simulink model "case4"  (R2024b)
settings: Solver=FixedStepAuto  StartTime=0  StopTime=1  FixedStep=1e-7  RelTol=1e-3
values from neighbouring files (symbols this model uses):
  SG_D_1_D = 0.01056    [IEEE9_case_parameters.m]    (also in case1_parameters.m; case2_parameters.m; case3_parameters.m; case4_parameters.m)
  SG_D_1_EnableSaturation = 0    [IEEE9_case_parameters.m]    (also in case1_parameters.m; case2_parameters.m; case3_parameters.m; case4_parameters.m)
  SG_D_1_f0 = 60    [IEEE9_case_parameters.m]    (also in case1_parameters.m; case2_parameters.m; case3_parameters.m; case4_parameters.m)
  SG_D_1_H = 7.5    [IEEE9_case_parameters.m]    (also in case1_parameters.m; case2_parameters.m; case3_parameters.m; case4_parameters.m)
  SG_D_1_K_A = 20    [IEEE9_case_parameters.m]    (also in case1_parameters.m; case2_parameters.m; case3_parameters.m; case4_parameters.m)
  SG_D_1_K_E = 1.000000e+1    (= 10)    [IEEE9_case_parameters.m]    (also in case1_parameters.m; case2_parameters.m; case3_parameters.m; case4_parameters.m)
  SG_D_1_K_F = 2.363    [IEEE9_case_parameters.m]    (also in case1_parameters.m; case2_parameters.m; case3_parameters.m; case4_parameters.m)
  SG_D_1_K_s = 0.5    [IEEE9_case_parameters.m]    (also in case1_parameters.m = 5; case2_parameters.m = 5; case3_parameters.m = 5; case4_parameters.m = 5)
  SG_D_1_R_a = 0.001088    [IEEE9_case_parameters.m]    (also in case1_parameters.m; case2_parameters.m; case3_parameters.m; case4_parameters.m)
  SG_D_1_S_A = 1    [IEEE9_case_parameters.m]    (also in case1_parameters.m; case2_parameters.m; case3_parameters.m; case4_parameters.m)
  SG_D_1_S_B = 0.103    [IEEE9_case_parameters.m]    (also in case1_parameters.m; case2_parameters.m; case3_parameters.m; case4_parameters.m)
  SG_D_1_S_N = 10.659857    [IEEE9_case_parameters.m]    (also in case1_parameters.m; case2_parameters.m; case3_parameters.m; case4_parameters.m)
  SG_D_1_SpeedPara = 200    [IEEE9_case_parameters.m]    (also in case1_parameters.m; case2_parameters.m; case3_parameters.m; case4_parameters.m)
  SG_D_1_T_0 = 0.720173    [IEEE9_case_parameters.m]    (also in case1_parameters.m = 0.755522; case2_parameters.m = 0.808931; case3_parameters.m = 0.869402; case4_parameters.m = 0.729316)
  SG_D_1_T_1 = 0.3    [IEEE9_case_parameters.m]    (also in case1_parameters.m; case2_parameters.m; case3_parameters.m; case4_parameters.m)
  SG_D_1_T_2 = 0.05    [IEEE9_case_parameters.m]    (also in case1_parameters.m; case2_parameters.m; case3_parameters.m; case4_parameters.m)
  SG_D_1_T_3 = 0.02    [IEEE9_case_parameters.m]    (also in case1_parameters.m; case2_parameters.m; case3_parameters.m; case4_parameters.m)
  SG_D_1_T_4 = 0.005    [IEEE9_case_parameters.m]    (also in case1_parameters.m; case2_parameters.m; case3_parameters.m; case4_parameters.m)
  SG_D_1_T_A = 0.02    [IEEE9_case_parameters.m]    (also in case1_parameters.m; case2_parameters.m; case3_parameters.m; case4_parameters.m)
  SG_D_1_T_dd = 8.000000e+0    (= 8)    [IEEE9_case_parameters.m]    (also in case1_parameters.m; case2_parameters.m; case3_parameters.m; case4_parameters.m)
  SG_D_1_T_ddd = 0.04    [IEEE9_case_parameters.m]    (also in case1_parameters.m; case2_parameters.m; case3_parameters.m; case4_parameters.m)
  SG_D_1_T_E = 0.314    [IEEE9_case_parameters.m]    (also in case1_parameters.m; case2_parameters.m; case3_parameters.m; case4_parameters.m)
  SG_D_1_T_F = 0.35    [IEEE9_case_parameters.m]    (also in case1_parameters.m; case2_parameters.m; case3_parameters.m; case4_parameters.m)
  SG_D_1_T_qd = 0.8    [IEEE9_case_parameters.m]    (also in case1_parameters.m; case2_parameters.m; case3_parameters.m; case4_parameters.m)
  SG_D_1_T_qdd = 0.02    [IEEE9_case_parameters.m]    (also in case1_parameters.m; case2_parameters.m; case3_parameters.m; case4_parameters.m)
  SG_D_1_T_speed = 0.1    [IEEE9_case_parameters.m]    (also in case1_parameters.m = 200; case2_parameters.m = 200; case3_parameters.m = 200; case4_parameters.m = 200)
  SG_D_1_T_w = 0.5    [IEEE9_case_parameters.m]    (also in case1_parameters.m; case2_parameters.m; case3_parameters.m; case4_parameters.m)
  SG_D_1_V_ref = 1.990276    [IEEE9_case_parameters.m]    (also in case1_parameters.m = 2.042296; case2_parameters.m = 2.051388; case3_parameters.m = 2.089584; case4_parameters.m = 2.01845)
  SG_D_1_w_ref = 376.991118    [IEEE9_case_parameters.m]    (also in case1_parameters.m; case2_parameters.m; case3_parameters.m; case4_parameters.m)
  SG_D_1_wb = 6.000000e+1    (= 60)    [IEEE9_case_parameters.m]    (also in case1_parameters.m; case2_parameters.m; case3_parameters.m; case4_parameters.m)
  SG_D_1_x_d = 1.9    [IEEE9_case_parameters.m]    (also in case1_parameters.m; case2_parameters.m; case3_parameters.m; case4_parameters.m)
  SG_D_1_x_dd = 0.302    [IEEE9_case_parameters.m]    (also in case1_parameters.m; case2_parameters.m; case3_parameters.m; case4_parameters.m)
  SG_D_1_x_ddd = 0.204    [IEEE9_case_parameters.m]    (also in case1_parameters.m; case2_parameters.m; case3_parameters.m; case4_parameters.m)
  SG_D_1_x_l = 0.05    [IEEE9_case_parameters.m]    (also in case1_parameters.m; case2_parameters.m; case3_parameters.m; case4_parameters.m)
  SG_D_1_x_q = 1.3    [IEEE9_case_parameters.m]    (also in case1_parameters.m; case2_parameters.m; case3_parameters.m; case4_parameters.m)
  SG_D_1_x_qd = 0.5    [IEEE9_case_parameters.m]    (also in case1_parameters.m; case2_parameters.m; case3_parameters.m; case4_parameters.m)
  SG_D_1_x_qdd = 0.3    [IEEE9_case_parameters.m]    (also in case1_parameters.m; case2_parameters.m; case3_parameters.m; case4_parameters.m)
  SG_D_2_D = 0.02    [IEEE9_case_parameters.m]    (also in case1_parameters.m; case2_parameters.m; case3_parameters.m; case4_parameters.m)
  SG_D_2_EnableSaturation = 0    [IEEE9_case_parameters.m]    (also in case1_parameters.m; case2_parameters.m; case3_parameters.m; case4_parameters.m)
  SG_D_2_f0 = 60    [IEEE9_case_parameters.m]    (also in case1_parameters.m; case2_parameters.m; case3_parameters.m; case4_parameters.m)
  SG_D_2_H = 8.000000e+0    (= 8)    [IEEE9_case_parameters.m]    (also in case1_parameters.m; case2_parameters.m; case3_parameters.m; case4_parameters.m)
  SG_D_2_K_A = 20    [IEEE9_case_parameters.m]    (also in case1_parameters.m; case2_parameters.m; case3_parameters.m; case4_parameters.m)
  SG_D_2_K_E = 1.000000e+1    (= 10)    [IEEE9_case_parameters.m]    (also in case1_parameters.m; case2_parameters.m; case3_parameters.m; case4_parameters.m)
  SG_D_2_K_F = 2.363    [IEEE9_case_parameters.m]    (also in case1_parameters.m; case2_parameters.m; case3_parameters.m; case4_parameters.m)
  SG_D_2_K_s = 0.5    [IEEE9_case_parameters.m]    (also in case1_parameters.m = 4; case2_parameters.m = 4; case3_parameters.m = 4; case4_parameters.m = 4)
  SG_D_2_R_a = 0.001088    [IEEE9_case_parameters.m]    (also in case1_parameters.m; case2_parameters.m; case3_parameters.m; case4_parameters.m)
  SG_D_2_S_A = 1    [IEEE9_case_parameters.m]    (also in case1_parameters.m; case2_parameters.m; case3_parameters.m; case4_parameters.m)
  SG_D_2_S_B = 0.103    [IEEE9_case_parameters.m]    (also in case1_parameters.m; case2_parameters.m; case3_parameters.m; case4_parameters.m)
  SG_D_2_S_N = 10.659857    [IEEE9_case_parameters.m]    (also in case1_parameters.m; case2_parameters.m; case3_parameters.m; case4_parameters.m)
  SG_D_2_SpeedPara = 200    [IEEE9_case_parameters.m]    (also in case1_parameters.m; case2_parameters.m; case3_parameters.m; case4_parameters.m)
  SG_D_2_T_0 = 1.632913    [IEEE9_case_parameters.m]    (also in case1_parameters.m = 1.632925; case2_parameters.m = 1.632915; case3_parameters.m = 1.632914; case4_parameters.m = 1.632927)
  SG_D_2_T_1 = 0.2    [IEEE9_case_parameters.m]    (also in case1_parameters.m; case2_parameters.m; case3_parameters.m; case4_parameters.m)
  SG_D_2_T_2 = 0.05    [IEEE9_case_parameters.m]    (also in case1_parameters.m; case2_parameters.m; case3_parameters.m; case4_parameters.m)
  SG_D_2_T_3 = 0.02    [IEEE9_case_parameters.m]    (also in case1_parameters.m; case2_parameters.m; case3_parameters.m; case4_parameters.m)
  SG_D_2_T_4 = 0.005    [IEEE9_case_parameters.m]    (also in case1_parameters.m; case2_parameters.m; case3_parameters.m; case4_parameters.m)
  SG_D_2_T_A = 0.02    [IEEE9_case_parameters.m]    (also in case1_parameters.m; case2_parameters.m; case3_parameters.m; case4_parameters.m)
  SG_D_2_T_dd = 7.9    [IEEE9_case_parameters.m]    (also in case1_parameters.m; case2_parameters.m; case3_parameters.m; case4_parameters.m)
  SG_D_2_T_ddd = 0.04    [IEEE9_case_parameters.m]    (also in case1_parameters.m; case2_parameters.m; case3_parameters.m; case4_parameters.m)
  SG_D_2_T_E = 0.314    [IEEE9_case_parameters.m]    (also in case1_parameters.m; case2_parameters.m; case3_parameters.m; case4_parameters.m)
  SG_D_2_T_F = 0.35    [IEEE9_case_parameters.m]    (also in case1_parameters.m; case2_parameters.m; case3_parameters.m; case4_parameters.m)
  SG_D_2_T_qd = 0.8    [IEEE9_case_parameters.m]    (also in case1_parameters.m; case2_parameters.m; case3_parameters.m; case4_parameters.m)
  SG_D_2_T_qdd = 0.015    [IEEE9_case_parameters.m]    (also in case1_parameters.m; case2_parameters.m; case3_parameters.m; case4_parameters.m)
  SG_D_2_T_speed = 0.1    [IEEE9_case_parameters.m]    (also in case1_parameters.m = 150; case2_parameters.m = 150; case3_parameters.m = 150; case4_parameters.m = 150)
  SG_D_2_T_w = 0.35    [IEEE9_case_parameters.m]    (also in case1_parameters.m; case2_parameters.m; case3_parameters.m; case4_parameters.m)
  SG_D_2_V_ref = 2.58547    [IEEE9_case_parameters.m]    (also in case1_parameters.m = 2.597896; case2_parameters.m = 2.587136; case3_parameters.m = 2.586042; case4_parameters.m = 2.599679)
  SG_D_2_w_ref = 376.991118    [IEEE9_case_parameters.m]    (also in case1_parameters.m; case2_parameters.m; case3_parameters.m; case4_parameters.m)
  SG_D_2_wb = 6.000000e+1    (= 60)    [IEEE9_case_parameters.m]    (also in case1_parameters.m; case2_parameters.m; case3_parameters.m; case4_parameters.m)
  SG_D_2_x_d = 1.8    [IEEE9_case_parameters.m]    (also in case1_parameters.m; case2_parameters.m; case3_parameters.m; case4_parameters.m)
  SG_D_2_x_dd = 0.302    [IEEE9_case_parameters.m]    (also in case1_parameters.m; case2_parameters.m; case3_parameters.m; case4_parameters.m)
  SG_D_2_x_ddd = 0.204    [IEEE9_case_parameters.m]    (also in case1_parameters.m; case2_parameters.m; case3_parameters.m; case4_parameters.m)
  SG_D_2_x_l = 0.05    [IEEE9_case_parameters.m]    (also in case1_parameters.m; case2_parameters.m; case3_parameters.m; case4_parameters.m)
  SG_D_2_x_q = 1.25    [IEEE9_case_parameters.m]    (also in case1_parameters.m; case2_parameters.m; case3_parameters.m; case4_parameters.m)
  SG_D_2_x_qd = 0.5    [IEEE9_case_parameters.m]    (also in case1_parameters.m; case2_parameters.m; case3_parameters.m; case4_parameters.m)
  SG_D_2_x_qdd = 0.3    [IEEE9_case_parameters.m]    (also in case1_parameters.m; case2_parameters.m; case3_parameters.m; case4_parameters.m)
  SG_D_3_D = 0.02    [IEEE9_case_parameters.m]    (also in case1_parameters.m; case2_parameters.m; case3_parameters.m; case4_parameters.m)
  SG_D_3_EnableSaturation = 0    [IEEE9_case_parameters.m]    (also in case1_parameters.m; case2_parameters.m; case3_parameters.m; case4_parameters.m)
  SG_D_3_f0 = 60    [IEEE9_case_parameters.m]    (also in case1_parameters.m; case2_parameters.m; case3_parameters.m; case4_parameters.m)
  SG_D_3_H = 7.7    [IEEE9_case_parameters.m]    (also in case1_parameters.m; case2_parameters.m; case3_parameters.m; case4_parameters.m)
  SG_D_3_K_A = 20    [IEEE9_case_parameters.m]    (also in case1_parameters.m; case2_parameters.m; case3_parameters.m; case4_parameters.m)
  SG_D_3_K_E = 1.000000e+1    (= 10)    [IEEE9_case_parameters.m]    (also in case1_parameters.m; case2_parameters.m; case3_parameters.m; case4_parameters.m)
  SG_D_3_K_F = 2.363    [IEEE9_case_parameters.m]    (also in case1_parameters.m; case2_parameters.m; case3_parameters.m; case4_parameters.m)
  SG_D_3_K_s = 0.2    [IEEE9_case_parameters.m]    (also in case1_parameters.m = 2; case2_parameters.m = 2; case3_parameters.m = 2; case4_parameters.m = 2)
  SG_D_3_R_a = 0.001088    [IEEE9_case_parameters.m]    (also in case1_parameters.m; case2_parameters.m; case3_parameters.m; case4_parameters.m)
  SG_D_3_S_A = 1    [IEEE9_case_parameters.m]    (also in case1_parameters.m; case2_parameters.m; case3_parameters.m; case4_parameters.m)
  SG_D_3_S_B = 0.103    [IEEE9_case_parameters.m]    (also in case1_parameters.m; case2_parameters.m; case3_parameters.m; case4_parameters.m)
  SG_D_3_S_N = 10.659857    [IEEE9_case_parameters.m]    (also in case1_parameters.m; case2_parameters.m; case3_parameters.m; case4_parameters.m)
  SG_D_3_SpeedPara = 200    [IEEE9_case_parameters.m]    (also in case1_parameters.m; case2_parameters.m; case3_parameters.m; case4_parameters.m)
  SG_D_3_T_0 = 0.850788    [IEEE9_case_parameters.m]    (also in case1_parameters.m = 0.850786; case2_parameters.m = 0.850787; case3_parameters.m; case4_parameters.m = 0.850786)
  SG_D_3_T_1 = 0.2    [IEEE9_case_parameters.m]    (also in case1_parameters.m; case2_parameters.m; case3_parameters.m; case4_parameters.m)
  SG_D_3_T_2 = 0.05    [IEEE9_case_parameters.m]    (also in case1_parameters.m; case2_parameters.m; case3_parameters.m; case4_parameters.m)
  SG_D_3_T_3 = 0.02    [IEEE9_case_parameters.m]    (also in case1_parameters.m; case2_parameters.m; case3_parameters.m; case4_parameters.m)
  SG_D_3_T_4 = 0.005    [IEEE9_case_parameters.m]    (also in case1_parameters.m; case2_parameters.m; case3_parameters.m; case4_parameters.m)
  SG_D_3_T_A = 0.02    [IEEE9_case_parameters.m]    (also in case1_parameters.m; case2_parameters.m; case3_parameters.m; case4_parameters.m)
  SG_D_3_T_dd = 8.1    [IEEE9_case_parameters.m]    (also in case1_parameters.m; case2_parameters.m; case3_parameters.m; case4_parameters.m)
  SG_D_3_T_ddd = 0.04    [IEEE9_case_parameters.m]    (also in case1_parameters.m; case2_parameters.m; case3_parameters.m; case4_parameters.m)
  SG_D_3_T_E = 0.314    [IEEE9_case_parameters.m]    (also in case1_parameters.m; case2_parameters.m; case3_parameters.m; case4_parameters.m)
  SG_D_3_T_F = 0.35    [IEEE9_case_parameters.m]    (also in case1_parameters.m; case2_parameters.m; case3_parameters.m; case4_parameters.m)
  SG_D_3_T_qd = 0.8    [IEEE9_case_parameters.m]    (also in case1_parameters.m; case2_parameters.m; case3_parameters.m; case4_parameters.m)
  SG_D_3_T_qdd = 0.015    [IEEE9_case_parameters.m]    (also in case1_parameters.m; case2_parameters.m; case3_parameters.m; case4_parameters.m)
  SG_D_3_T_speed = 0.1    [IEEE9_case_parameters.m]    (also in case1_parameters.m = 180; case2_parameters.m = 180; case3_parameters.m = 180; case4_parameters.m = 180)
  SG_D_3_T_w = 0.4    [IEEE9_case_parameters.m]    (also in case1_parameters.m; case2_parameters.m; case3_parameters.m; case4_parameters.m)
  SG_D_3_V_ref = 1.892727    [IEEE9_case_parameters.m]    (also in case1_parameters.m = 1.906439; case2_parameters.m = 1.895535; case3_parameters.m = 1.892105; case4_parameters.m = 1.906598)
  SG_D_3_w_ref = 376.991118    [IEEE9_case_parameters.m]    (also in case1_parameters.m; case2_parameters.m; case3_parameters.m; case4_parameters.m)
  SG_D_3_wb = 6.000000e+1    (= 60)    [IEEE9_case_parameters.m]    (also in case1_parameters.m; case2_parameters.m; case3_parameters.m; case4_parameters.m)
  SG_D_3_x_d = 1.85    [IEEE9_case_parameters.m]    (also in case1_parameters.m; case2_parameters.m; case3_parameters.m; case4_parameters.m)
  SG_D_3_x_dd = 0.302    [IEEE9_case_parameters.m]    (also in case1_parameters.m; case2_parameters.m; case3_parameters.m; case4_parameters.m)
  SG_D_3_x_ddd = 0.204    [IEEE9_case_parameters.m]    (also in case1_parameters.m; case2_parameters.m; case3_parameters.m; case4_parameters.m)
  SG_D_3_x_l = 0.05    [IEEE9_case_parameters.m]    (also in case1_parameters.m; case2_parameters.m; case3_parameters.m; case4_parameters.m)
  SG_D_3_x_q = 1.2    [IEEE9_case_parameters.m]    (also in case1_parameters.m; case2_parameters.m; case3_parameters.m; case4_parameters.m)
  SG_D_3_x_qd = 0.5    [IEEE9_case_parameters.m]    (also in case1_parameters.m; case2_parameters.m; case3_parameters.m; case4_parameters.m)
  SG_D_3_x_qdd = 0.3    [IEEE9_case_parameters.m]    (also in case1_parameters.m; case2_parameters.m; case3_parameters.m; case4_parameters.m)
(part 5 of 12)

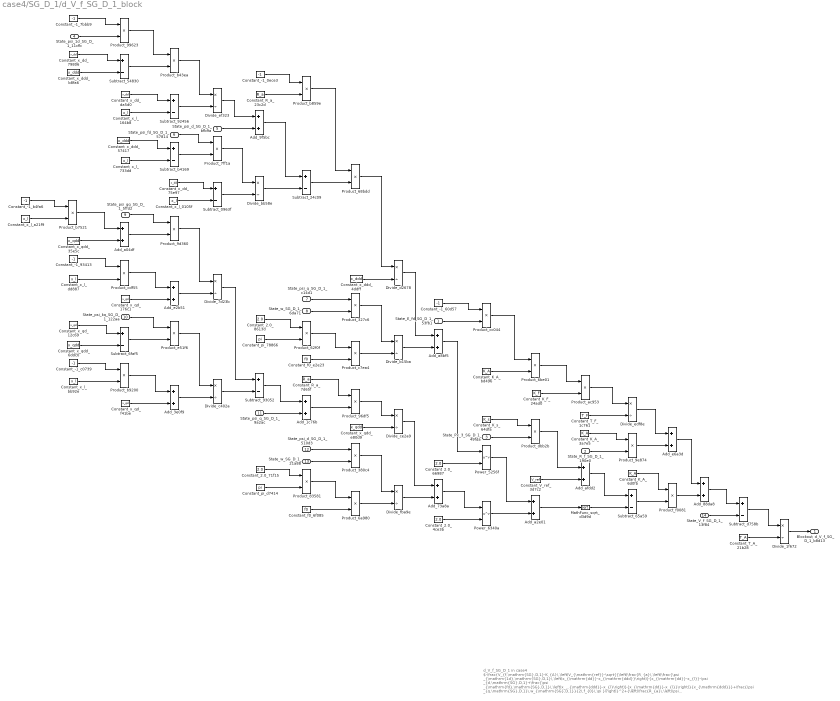
== system case4/SG_D_1/d_V_f_SG_D_1_block ==
  note: d_V_f_SG_D_1 in case4
      | $-\frac{V_{f,\mathrm{SG},D,1}-K_{A}\,\left(V_{\mathrm{ref}}-\sqrt{{\left(\frac{R_{a}\,\left(\frac{\psi _{\mathrm{1d},\mathrm{SG},D,1}\,\left(x_{\mathrm{dd}}-x_{\mathrm{ddd}}\right)}{x_{\mathrm{dd}}-x_{l}}-\psi _{d,\mathrm{SG},D,1}+\frac{\psi _{\mathrm{fd},\mathrm{SG},D,1}\,\left(x_{\mathrm{ddd}}-x_{l}\right)}{x_{\mathrm{dd}}-x_{l}}\right)}{x_{\mathrm{ddd}}}+\frac{\psi _{q,\mathrm{SG},D,1}\,w_{\mathrm{SG},D,1}}{2\,f_{0}\,\pi }\right)}^2+{\left(\frac{R_{a}\,\left(\psi _{q,\mathrm{SG},D,1}+\frac{\psi _{\mathrm{gq},\mathrm{SG},D,1}\,\left(x_{l}-x_{\mathrm{qdd}}\right)}{x_{l}-x_{\mathrm{qd}}}+\frac{\psi _{\mathrm{kq},\mathrm{SG},D,1}\,\left(x_{\mathrm{qd}}-x_{\mathrm{qdd}}\right)}{x_{l}-x_{\mathrm{qd}}}\right)}{x_{\mathrm{qdd}}}+\frac{\psi _{d,\mathrm{SG},D,1}\,w_{\mathrm{SG},D,1}}{2\,f_{0}\,\pi }\right)}^2}+K_{s}\,\mathrm{Px}_{3,\mathrm{SG},D,1}\right)-K_{A}\,R_{f,\mathrm{SG},D,1}+\frac{E_{\mathrm{fd},\mathrm{SG},D,1}\,K_{A}\,K_{F}}{T_{F}}}{T_{A}}$
      | Automatically generated on 2025-10-31 19:04:43 .
  State_E_fd_SG_D_1_53fb1 : Inport
  State_R_f_SG_D_1_190e0 : Inport  Port=2
  State_Px_3_SG_D_1_49fda : Inport  Port=3
  State_psi_1d_SG_D_1_11cfb : Inport  Port=4
  State_psi_d_SG_D_1_bfb9a : Inport  Port=5
  State_psi_fd_SG_D_1_57814 : Inport  Port=6
  State_psi_q_SG_D_1_c14d1 : Inport  Port=7
  State_w_SG_D_1_6da71 : Inport  Port=8
  State_psi_gq_SG_D_1_5ffd2 : Inport  Port=9
  State_psi_kq_SG_D_1_122aa : Inport  Port=10
  State_psi_q_SG_D_1_9a2ac : Inport  Port=11
  State_psi_d_SG_D_1_510d3 : Inport  Port=12
  State_w_SG_D_1_21a88 : Inport  Port=13
  State_V_f_SG_D_1_13f84 : Inport  Port=14
  Add_1c76b : Sum
  Add_3e0f9 : Sum
  Add_73a8a : Sum
  Add_88da8 : Sum
  Add_9f5bc : Sum
  Add_a04df : Sum
  Add_a2e01 : Sum
  Add_a8bf5 : Sum
  Add_afdd2 : Sum
  Add_e2b51 : Sum
  Add_e6a3d : Sum
  Constant_-1_0ece3 : Constant  Value=-1
  Constant_-1_60d57 : Constant  Value=-1
  Constant_-1_7bbb9 : Constant  Value=-1
  Constant_-1_93413 : Constant  Value=-1
  Constant_-1_b4fa6 : Constant  Value=-1
  Constant_-1_c0739 : Constant  Value=-1
  Constant_2.0_4ce3b : Constant  Value=2.0
  Constant_2.0_66987 : Constant  Value=2.0
  Constant_2.0_71f15 : Constant  Value=2.0
  Constant_2.0_8613d : Constant  Value=2.0
  Constant_K_A_3a7e5 : Constant  Value=K_A
  Constant_K_A_6d0fb : Constant  Value=K_A
  Constant_K_A_bd496 : Constant  Value=K_A
  Constant_K_F_24ad0 : Constant  Value=K_F
  Constant_K_s_64dfa : Constant  Value=K_s
  Constant_R_a_23c2d : Constant  Value=R_a
  Constant_R_a_7d65f : Constant  Value=R_a
  Constant_T_A_21b28 : Constant  Value=T_A
  Constant_T_F_1c761 : Constant  Value=T_F
  Constant_V_ref_3d7c2 : Constant  Value=V_ref
  Constant_f0_6f085 : Constant  Value=f0
  Constant_f0_e2e23 : Constant  Value=f0
  Constant_pi_78866 : Constant  Value=pi
  Constant_pi_d7414 : Constant  Value=pi
  Constant_x_dd_75e97 : Constant  Value=x_dd
  Constant_x_dd_79806 : Constant  Value=x_dd
  Constant_x_dd_da5d0 : Constant  Value=x_dd
  Constant_x_ddd_4ddff : Constant  Value=x_ddd
  Constant_x_ddd_57417 : Constant  Value=x_ddd
  Constant_x_ddd_b8fa6 : Constant  Value=x_ddd
  Constant_x_l_0105f : Constant  Value=x_l
  Constant_x_l_164b8 : Constant  Value=x_l
  Constant_x_l_733dd : Constant  Value=x_l
  Constant_x_l_a21f9 : Constant  Value=x_l
  Constant_x_l_bb92e : Constant  Value=x_l
  Constant_x_l_dd887 : Constant  Value=x_l
  Constant_x_qd_12c69 : Constant  Value=x_qd
  Constant_x_qd_176c1 : Constant  Value=x_qd
  Constant_x_qd_f41be : Constant  Value=x_qd
  Constant_x_qdd_35e5c : Constant  Value=x_qdd
  Constant_x_qdd_6ddc0 : Constant  Value=x_qdd
  Constant_x_qdd_e80d9 : Constant  Value=x_qdd
  Divide_1f672 : Product  Inputs=*/
  Divide_7d23b : Product  Inputs=*/
  Divide_b15ba : Product  Inputs=*/
  Divide_bb58e : Product  Inputs=*/
  Divide_c402a : Product  Inputs=*/
  Divide_ce2a9 : Product  Inputs=*/
  Divide_d2678 : Product  Inputs=*/
  Divide_edf8e : Product  Inputs=*/
  Divide_ef323 : Product  Inputs=*/
  Divide_fba9e : Product  Inputs=*/
  MathFunc_sqrt_d3d9d : Sqrt
  Power_5256f : Math  Operator=pow
  Power_6340a : Math  Operator=pow
  Product_327c6 : Product
  Product_380c4 : Product
  Product_62f0f : Product
  Product_68bdd : Product
  Product_6a980 : Product
  Product_6be01 : Product
  Product_7ff1a : Product
  Product_83581 : Product
  Product_96df5 : Product
  Product_99623 : Product
  Product_9d360 : Product
  Product_9e874 : Product
  Product_ac953 : Product
  Product_b43ea : Product
  Product_b7521 : Product
  Product_b859e : Product
  Product_b9200 : Product
  Product_c7ea4 : Product
  Product_cc044 : Product
  Product_cdf55 : Product
  Product_dbb2b : Product
  Product_e51f6 : Product
  Product_f0081 : Product
  Subtract_0963f : Sum  Inputs=+-
  Subtract_24c09 : Sum  Inputs=+-
  Subtract_54830 : Sum  Inputs=+-
  Subtract_65a59 : Sum  Inputs=+-
  Subtract_6faf5 : Sum  Inputs=+-
  Subtract_92456 : Sum  Inputs=+-
  Subtract_93052 : Sum  Inputs=+-
  Subtract_b4169 : Sum  Inputs=+-
  Subtract_d758b : Sum  Inputs=+-
  Blockout_d_V_f_SG_D_1_b8d13 : Outport
  wires:
  Constant_-1_c0739/1 -> Product_b9200/1
  Constant_-1_b4fa6/1 -> Product_b7521/1
  State_psi_d_SG_D_1_510d3/1 -> Product_380c4/1
  Constant_x_qd_f41be/1 -> Add_3e0f9/2
  Constant_x_qdd_35e5c/1 -> Add_a04df/2
  State_w_SG_D_1_21a88/1 -> Product_380c4/2
  Constant_x_l_a21f9/1 -> Product_b7521/2
  Subtract_24c09/1 -> Product_68bdd/2
  Constant_x_l_bb92e/1 -> Product_b9200/2
  Constant_x_dd_79806/1 -> Subtract_54830/1
  Constant_R_a_23c2d/1 -> Product_b859e/2
  Constant_-1_7bbb9/1 -> Product_99623/1
  Divide_bb58e/1 -> Subtract_24c09/2
  Constant_x_ddd_b8fa6/1 -> Subtract_54830/2
  Add_3e0f9/1 -> Divide_c402a/2
  State_psi_1d_SG_D_1_11cfb/1 -> Product_99623/2
  Add_e2b51/1 -> Divide_7d23b/2
  Subtract_6faf5/1 -> Product_e51f6/2
  Product_ac953/1 -> Divide_edf8e/1
  Product_62f0f/1 -> Product_c7ea4/1
  Product_b7521/1 -> Add_a04df/1
  Constant_-1_93413/1 -> Product_cdf55/1
  Constant_x_l_dd887/1 -> Product_cdf55/2
  Add_9f5bc/1 -> Subtract_24c09/1
  Constant_2.0_71f15/1 -> Product_83581/1
  Constant_x_qd_12c69/1 -> Subtract_6faf5/1
  Product_99623/1 -> Product_b43ea/1
  Constant_pi_d7414/1 -> Product_83581/2
  Constant_x_qdd_6ddc0/1 -> Subtract_6faf5/2
  Subtract_54830/1 -> Product_b43ea/2
  State_psi_q_SG_D_1_9a2ac/1 -> Add_1c76b/2
  Constant_x_dd_da5d0/1 -> Subtract_92456/1
  Constant_x_l_164b8/1 -> Subtract_92456/2
  Constant_x_ddd_57417/1 -> Subtract_b4169/1
  Constant_x_l_733dd/1 -> Subtract_b4169/2
  State_psi_gq_SG_D_1_5ffd2/1 -> Product_9d360/1
  Add_a04df/1 -> Product_9d360/2
  Product_cdf55/1 -> Add_e2b51/1
  Constant_x_qd_176c1/1 -> Add_e2b51/2
  Divide_ef323/1 -> Add_9f5bc/1
  Subtract_92456/1 -> Divide_ef323/2
  State_psi_kq_SG_D_1_122aa/1 -> Product_e51f6/1
  Divide_1f672/1 -> Blockout_d_V_f_SG_D_1_b8d13/1
  Product_b9200/1 -> Add_3e0f9/1
  Product_b43ea/1 -> Divide_ef323/1
  State_psi_fd_SG_D_1_57814/1 -> Product_7ff1a/1
  State_w_SG_D_1_6da71/1 -> Product_327c6/2
  Subtract_b4169/1 -> Product_7ff1a/2
  Constant_x_dd_75e97/1 -> Subtract_0963f/1
  Constant_x_l_0105f/1 -> Subtract_0963f/2
  Product_9d360/1 -> Divide_7d23b/1
  Product_b859e/1 -> Product_68bdd/1
  Product_e51f6/1 -> Divide_c402a/1
  State_psi_d_SG_D_1_bfb9a/1 -> Add_9f5bc/2
  Product_7ff1a/1 -> Divide_bb58e/1
  Subtract_0963f/1 -> Divide_bb58e/2
  Divide_7d23b/1 -> Subtract_93052/1
  Divide_c402a/1 -> Subtract_93052/2
  Constant_-1_0ece3/1 -> Product_b859e/1
  Constant_2.0_8613d/1 -> Product_62f0f/1
  Constant_pi_78866/1 -> Product_62f0f/2
  Subtract_93052/1 -> Add_1c76b/1
  State_psi_q_SG_D_1_c14d1/1 -> Product_327c6/1
  Constant_f0_e2e23/1 -> Product_c7ea4/2
  Constant_R_a_7d65f/1 -> Product_96df5/1
  Add_1c76b/1 -> Product_96df5/2
  Product_83581/1 -> Product_6a980/1
  Power_5256f/1 -> Add_a2e01/1
  Constant_f0_6f085/1 -> Product_6a980/2
  Product_68bdd/1 -> Divide_d2678/1
  Constant_x_ddd_4ddff/1 -> Divide_d2678/2
  Product_327c6/1 -> Divide_b15ba/1
  Product_c7ea4/1 -> Divide_b15ba/2
  Product_96df5/1 -> Divide_ce2a9/1
  Constant_x_qdd_e80d9/1 -> Divide_ce2a9/2
  Product_380c4/1 -> Divide_fba9e/1
  Product_6a980/1 -> Divide_fba9e/2
  Divide_d2678/1 -> Add_a8bf5/1
  Divide_b15ba/1 -> Add_a8bf5/2
  Divide_ce2a9/1 -> Add_73a8a/1
  Divide_fba9e/1 -> Add_73a8a/2
  Constant_-1_60d57/1 -> Product_cc044/1
  State_E_fd_SG_D_1_53fb1/1 -> Product_cc044/2
  Add_a8bf5/1 -> Power_5256f/1
  Constant_2.0_66987/1 -> Power_5256f/2
  Add_73a8a/1 -> Power_6340a/1
  Constant_2.0_4ce3b/1 -> Power_6340a/2
  Product_cc044/1 -> Product_6be01/1
  Constant_K_A_bd496/1 -> Product_6be01/2
  Constant_K_s_64dfa/1 -> Product_dbb2b/1
  State_Px_3_SG_D_1_49fda/1 -> Product_dbb2b/2
  Power_6340a/1 -> Add_a2e01/2
  Divide_edf8e/1 -> Add_e6a3d/1
  Product_6be01/1 -> Product_ac953/1
  Constant_K_F_24ad0/1 -> Product_ac953/2
  Product_dbb2b/1 -> Add_afdd2/1
  Constant_V_ref_3d7c2/1 -> Add_afdd2/2
  Add_a2e01/1 -> MathFunc_sqrt_d3d9d/1
  Constant_T_F_1c761/1 -> Divide_edf8e/2
  Constant_K_A_3a7e5/1 -> Product_9e874/1
  State_R_f_SG_D_1_190e0/1 -> Product_9e874/2
  Add_afdd2/1 -> Subtract_65a59/1
  MathFunc_sqrt_d3d9d/1 -> Subtract_65a59/2
  Constant_T_A_21b28/1 -> Divide_1f672/2
  Product_9e874/1 -> Add_e6a3d/2
  Constant_K_A_6d0fb/1 -> Product_f0081/1
  Subtract_65a59/1 -> Product_f0081/2
  Add_e6a3d/1 -> Add_88da8/1
  Product_f0081/1 -> Add_88da8/2
  Add_88da8/1 -> Subtract_d758b/1
  State_V_f_SG_D_1_13f84/1 -> Subtract_d758b/2
  Subtract_d758b/1 -> Divide_1f672/1

== system case4/SG_D_1/d_psi_1d_SG_D_1_block ==
  note: d_psi_1d_SG_D_1 in case4
      | $-\frac{\psi _{\mathrm{1d},\mathrm{SG},D,1}-\psi _{\mathrm{fd},\mathrm{SG},D,1}+\frac{\left(x_{\mathrm{dd}}-x_{l}\right)\,\left(\frac{\psi _{\mathrm{1d},\mathrm{SG},D,1}\,\left(x_{\mathrm{dd}}-x_{\mathrm{ddd}}\right)}{x_{\mathrm{dd}}-x_{l}}-\psi _{d,\mathrm{SG},D,1}+\frac{\psi _{\mathrm{fd},\mathrm{SG},D,1}\,\left(x_{\mathrm{ddd}}-x_{l}\right)}{x_{\mathrm{dd}}-x_{l}}\right)}{x_{\mathrm{ddd}}}}{T_{\mathrm{ddd}}}$
      | Automatically generated on 2025-10-31 19:04:18 .
  State_psi_1d_SG_D_1_22eb8 : Inport
  State_psi_fd_SG_D_1_06852 : Inport  Port=2
  State_psi_1d_SG_D_1_92ecb : Inport  Port=3
  State_psi_d_SG_D_1_6d1a3 : Inport  Port=4
  State_psi_fd_SG_D_1_52850 : Inport  Port=5
  Add_1f352 : Sum
  Add_32c2e : Sum
  Add_b799e : Sum
  Constant_-1_7fa6f : Constant  Value=-1
  Constant_-1_f3dc6 : Constant  Value=-1
  Constant_T_ddd_376ae : Constant  Value=T_ddd
  Constant_x_dd_12505 : Constant  Value=x_dd
  Constant_x_dd_39702 : Constant  Value=x_dd
  Constant_x_dd_3ec7f : Constant  Value=x_dd
  Constant_x_dd_f690e : Constant  Value=x_dd
  Constant_x_ddd_2ccd5 : Constant  Value=x_ddd
  Constant_x_ddd_39764 : Constant  Value=x_ddd
  Constant_x_ddd_f1a74 : Constant  Value=x_ddd
  Constant_x_l_1c7d9 : Constant  Value=x_l
  Constant_x_l_2bb5f : Constant  Value=x_l
  Constant_x_l_579c4 : Constant  Value=x_l
  Constant_x_l_f7cad : Constant  Value=x_l
  Divide_64f14 : Product  Inputs=*/
  Divide_7cf09 : Product  Inputs=*/
  Divide_a5915 : Product  Inputs=*/
  Divide_f4ab9 : Product  Inputs=*/
  Product_3bd75 : Product
  Product_46273 : Product
  Product_e0514 : Product
  Product_e1a7d : Product
  Product_f4c5c : Product
  Subtract_15020 : Sum  Inputs=+-
  Subtract_1a4ca : Sum  Inputs=+-
  Subtract_3ddd7 : Sum  Inputs=+-
  Subtract_49694 : Sum  Inputs=+-
  Subtract_8605b : Sum  Inputs=+-
  Subtract_e68a2 : Sum  Inputs=+-
  Blockout_d_psi_1d_SG_D_1_4f588 : Outport
  wires:
  Product_f4c5c/1 -> Product_e0514/1
  Constant_-1_f3dc6/1 -> Product_f4c5c/1
  Subtract_3ddd7/1 -> Product_e0514/2
  State_psi_1d_SG_D_1_92ecb/1 -> Product_f4c5c/2
  Subtract_1a4ca/1 -> Product_e1a7d/1
  State_psi_d_SG_D_1_6d1a3/1 -> Add_1f352/2
  Constant_x_dd_f690e/1 -> Subtract_49694/1
  Constant_x_l_1c7d9/1 -> Subtract_1a4ca/2
  Constant_x_dd_39702/1 -> Subtract_3ddd7/1
  Subtract_8605b/1 -> Product_46273/2
  Constant_x_l_2bb5f/1 -> Subtract_49694/2
  Divide_7cf09/1 -> Subtract_15020/2
  Constant_x_ddd_2ccd5/1 -> Subtract_3ddd7/2
  Constant_x_ddd_f1a74/1 -> Subtract_8605b/1
  Constant_x_l_579c4/1 -> Subtract_8605b/2
  Add_b799e/1 -> Add_32c2e/1
  Product_e0514/1 -> Divide_f4ab9/1
  Divide_64f14/1 -> Add_32c2e/2
  Subtract_49694/1 -> Divide_f4ab9/2
  State_psi_fd_SG_D_1_52850/1 -> Product_46273/1
  Constant_x_dd_3ec7f/1 -> Subtract_e68a2/1
  Constant_x_l_f7cad/1 -> Subtract_e68a2/2
  Constant_x_ddd_39764/1 -> Divide_64f14/2
  Subtract_15020/1 -> Product_e1a7d/2
  Divide_f4ab9/1 -> Add_1f352/1
  Product_46273/1 -> Divide_7cf09/1
  Subtract_e68a2/1 -> Divide_7cf09/2
  Product_e1a7d/1 -> Divide_64f14/1
  Constant_x_dd_12505/1 -> Subtract_1a4ca/1
  Add_1f352/1 -> Subtract_15020/1
  Constant_-1_7fa6f/1 -> Product_3bd75/1
  State_psi_1d_SG_D_1_22eb8/1 -> Product_3bd75/2
  Product_3bd75/1 -> Add_b799e/1
  State_psi_fd_SG_D_1_06852/1 -> Add_b799e/2
  Add_32c2e/1 -> Divide_a5915/1
  Constant_T_ddd_376ae/1 -> Divide_a5915/2
  Divide_a5915/1 -> Blockout_d_psi_1d_SG_D_1_4f588/1

== system case4/SG_D_1/d_psi_d_SG_D_1_block ==
  note: d_psi_d_SG_D_1 in case4
      | $2\,\pi \,f_{0}\,\left(v_{d,\mathrm{SG},D,1}\,\sin\left(\theta _{\mathrm{SG},D,1}\right)-v_{q,\mathrm{SG},D,1}\,\cos\left(\theta _{\mathrm{SG},D,1}\right)+\frac{R_{a}\,\left(\frac{\psi _{\mathrm{1d},\mathrm{SG},D,1}\,\left(x_{\mathrm{dd}}-x_{\mathrm{ddd}}\right)}{x_{\mathrm{dd}}-x_{l}}-\psi _{d,\mathrm{SG},D,1}+\frac{\psi _{\mathrm{fd},\mathrm{SG},D,1}\,\left(x_{\mathrm{ddd}}-x_{l}\right)}{x_{\mathrm{dd}}-x_{l}}\right)}{x_{\mathrm{ddd}}}+\frac{\psi _{q,\mathrm{SG},D,1}\,w_{\mathrm{SG},D,1}}{2\,f_{0}\,\pi }\right)$
      | Automatically generated on 2025-10-31 19:03:53 .
  State_psi_1d_SG_D_1_2ee34 : Inport
  State_psi_d_SG_D_1_3993f : Inport  Port=2
  State_psi_fd_SG_D_1_8a26a : Inport  Port=3
  Input_v_d_SG_D_1_2ca50 : Inport  Port=4
  State_theta_SG_D_1_ccf09 : Inport  Port=5
  Input_v_q_SG_D_1_1e814 : Inport  Port=6
  State_theta_SG_D_1_4ed89 : Inport  Port=7
  State_psi_q_SG_D_1_1479a : Inport  Port=8
  State_w_SG_D_1_d3493 : Inport  Port=9
  Add_096ff : Sum
  Add_49165 : Sum
  Constant_-1_1af36 : Constant  Value=-1
  Constant_-2.0_080a3 : Constant  Value=-2.0
  Constant_2.0_2e70a : Constant  Value=2.0
  Constant_R_a_e898f : Constant  Value=R_a
  Constant_f0_1e7bd : Constant  Value=f0
  Constant_f0_4f825 : Constant  Value=f0
  Constant_pi_2675e : Constant  Value=pi
  Constant_pi_9283c : Constant  Value=pi
  Constant_x_dd_02c26 : Constant  Value=x_dd
  Constant_x_dd_9050a : Constant  Value=x_dd
  Constant_x_dd_d1e50 : Constant  Value=x_dd
  Constant_x_ddd_64ab5 : Constant  Value=x_ddd
  Constant_x_ddd_adcef : Constant  Value=x_ddd
  Constant_x_ddd_fa74c : Constant  Value=x_ddd
  Constant_x_l_1327e : Constant  Value=x_l
  Constant_x_l_5f2ed : Constant  Value=x_l
  Constant_x_l_c2992 : Constant  Value=x_l
  Divide_3642b : Product  Inputs=*/
  Divide_88783 : Product  Inputs=*/
  Divide_ab901 : Product  Inputs=*/
  Divide_dfc10 : Product  Inputs=*/
  MathFunc_cos_0d94f : Trigonometry  Operator=cos
  MathFunc_sin_b6279 : Trigonometry
  Product_007ac : Product
  Product_01181 : Product
  Product_703dd : Product
  Product_95912 : Product
  Product_9e695 : Product
  Product_a4fd0 : Product
  Product_b0f24 : Product
  Product_b2b5d : Product
  Product_d773a : Product
  Product_e41ea : Product
  Product_f144a : Product
  Product_ffc8f : Product
  Subtract_110d4 : Sum  Inputs=+-
  Subtract_1642e : Sum  Inputs=+-
  Subtract_87af6 : Sum  Inputs=+-
  Subtract_8c989 : Sum  Inputs=+-
  Subtract_90b39 : Sum  Inputs=+-
  Subtract_931f4 : Sum  Inputs=+-
  Subtract_be43e : Sum  Inputs=+-
  Blockout_d_psi_d_SG_D_1_83a0e : Outport
  wires:
  Add_49165/1 -> Subtract_110d4/1
  Product_b2b5d/1 -> Divide_dfc10/1
  Subtract_87af6/1 -> Product_b2b5d/2
  Divide_dfc10/1 -> Add_49165/1
  Product_01181/1 -> Product_b2b5d/1
  Constant_x_ddd_fa74c/1 -> Subtract_87af6/2
  Constant_x_dd_9050a/1 -> Subtract_87af6/1
  State_psi_1d_SG_D_1_2ee34/1 -> Product_01181/2
  Constant_-1_1af36/1 -> Product_01181/1
  Product_703dd/1 -> Divide_88783/1
  Constant_x_l_5f2ed/1 -> Subtract_931f4/2
  State_psi_d_SG_D_1_3993f/1 -> Add_49165/2
  Constant_x_dd_02c26/1 -> Subtract_931f4/1
  Constant_x_ddd_adcef/1 -> Subtract_be43e/1
  Constant_x_l_1327e/1 -> Subtract_be43e/2
  Subtract_931f4/1 -> Divide_dfc10/2
  State_psi_fd_SG_D_1_8a26a/1 -> Product_703dd/1
  Constant_x_ddd_64ab5/1 -> Divide_ab901/2
  Subtract_be43e/1 -> Product_703dd/2
  Product_b0f24/1 -> Subtract_90b39/2
  Constant_x_dd_d1e50/1 -> Subtract_8c989/1
  Constant_x_l_c2992/1 -> Subtract_8c989/2
  Subtract_8c989/1 -> Divide_88783/2
  Divide_88783/1 -> Subtract_110d4/2
  Constant_R_a_e898f/1 -> Product_95912/1
  Subtract_110d4/1 -> Product_95912/2
  MathFunc_cos_0d94f/1 -> Product_9e695/2
  State_theta_SG_D_1_ccf09/1 -> MathFunc_sin_b6279/1
  Divide_ab901/1 -> Subtract_90b39/1
  Product_95912/1 -> Divide_ab901/1
  MathFunc_sin_b6279/1 -> Product_b0f24/2
  Input_v_d_SG_D_1_2ca50/1 -> Product_b0f24/1
  Product_d773a/1 -> Blockout_d_psi_d_SG_D_1_83a0e/1
  Product_007ac/1 -> Product_d773a/1
  Product_ffc8f/1 -> Product_007ac/1
  State_theta_SG_D_1_4ed89/1 -> MathFunc_cos_0d94f/1
  Constant_2.0_2e70a/1 -> Product_f144a/1
  Constant_pi_2675e/1 -> Product_f144a/2
  Input_v_q_SG_D_1_1e814/1 -> Product_9e695/1
  Constant_f0_1e7bd/1 -> Product_007ac/2
  State_psi_q_SG_D_1_1479a/1 -> Product_a4fd0/1
  State_w_SG_D_1_d3493/1 -> Product_a4fd0/2
  Product_f144a/1 -> Product_e41ea/1
  Constant_pi_9283c/1 -> Product_ffc8f/2
  Constant_f0_4f825/1 -> Product_e41ea/2
  Constant_-2.0_080a3/1 -> Product_ffc8f/1
  Add_096ff/1 -> Subtract_1642e/1
  Subtract_90b39/1 -> Add_096ff/1
  Product_9e695/1 -> Add_096ff/2
  Product_a4fd0/1 -> Divide_3642b/1
  Product_e41ea/1 -> Divide_3642b/2
  Divide_3642b/1 -> Subtract_1642e/2
  Subtract_1642e/1 -> Product_d773a/2

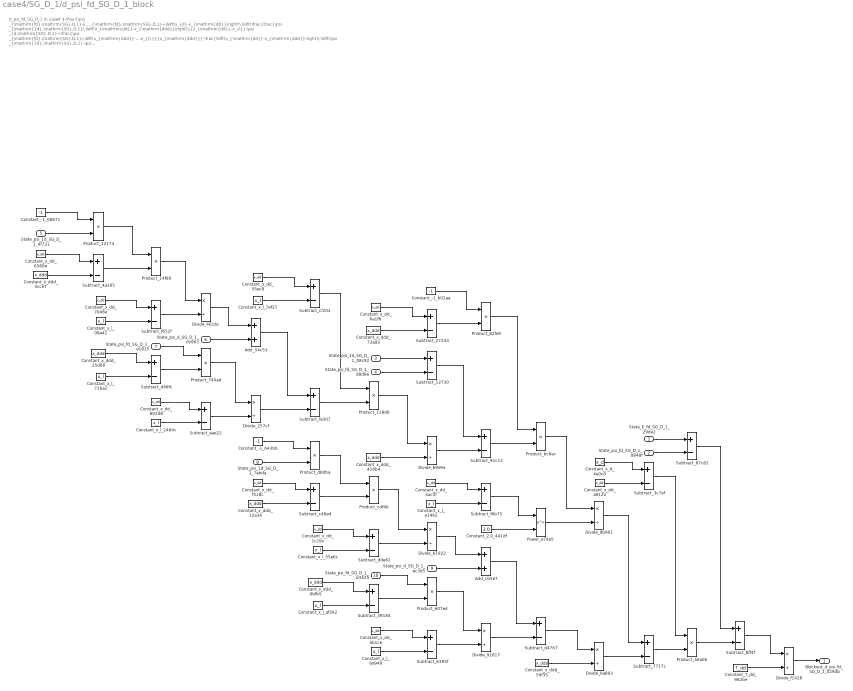
== system case4/SG_D_1/d_psi_fd_SG_D_1_block ==
  note: d_psi_fd_SG_D_1 in case4
      | $-\frac{\psi _{\mathrm{fd},\mathrm{SG},D,1}-E_{\mathrm{fd},\mathrm{SG},D,1}+\left(x_{d}-x_{\mathrm{dd}}\right)\,\left(\frac{\frac{\psi _{\mathrm{1d},\mathrm{SG},D,1}\,\left(x_{\mathrm{dd}}-x_{\mathrm{ddd}}\right)}{x_{\mathrm{dd}}-x_{l}}-\psi _{d,\mathrm{SG},D,1}+\frac{\psi _{\mathrm{fd},\mathrm{SG},D,1}\,\left(x_{\mathrm{ddd}}-x_{l}\right)}{x_{\mathrm{dd}}-x_{l}}}{x_{\mathrm{ddd}}}-\frac{\left(x_{\mathrm{dd}}-x_{\mathrm{ddd}}\right)\,\left(\psi _{\mathrm{1d},\mathrm{SG},D,1}-\psi _{\mathrm{fd},\mathrm{SG},D,1}+\frac{\left(x_{\mathrm{dd}}-x_{l}\right)\,\left(\frac{\psi _{\mathrm{1d},\mathrm{SG},D,1}\,\left(x_{\mathrm{dd}}-x_{\mathrm{ddd}}\right)}{x_{\mathrm{dd}}-x_{l}}-\psi _{d,\mathrm{SG},D,1}+\frac{\psi _{\mathrm{fd},\mathrm{SG},D,1}\,\left(x_{\mathrm{ddd}}-x_{l}\right)}{x_{\mathrm{dd}}-x_{l}}\right)}{x_{\mathrm{ddd}}}\right)}{{\left(x_{\mathrm{dd}}-x_{l}\right)}^2}\right)}{T_{\mathrm{dd}}}$
      | Automatically generated on 2025-10-31 19:04:15 .
  State_E_fd_SG_D_1_29de2 : Inport
  State_psi_fd_SG_D_1_0848f : Inport  Port=2
  State_psi_1d_SG_D_1_08c92 : Inport  Port=3
  State_psi_fd_SG_D_1_d8d8e : Inport  Port=4
  State_psi_1d_SG_D_1_4f731 : Inport  Port=5
  State_psi_d_SG_D_1_cb963 : Inport  Port=6
  State_psi_fd_SG_D_1_e1815 : Inport  Port=7
  State_psi_1d_SG_D_1_7ebda : Inport  Port=8
  State_psi_d_SG_D_1_ec3d5 : Inport  Port=9
  State_psi_fd_SG_D_1_d3425 : Inport  Port=10
  Add_54c53 : Sum
  Add_cb5e7 : Sum
  Constant_-1_08871 : Constant  Value=-1
  Constant_-1_643bb : Constant  Value=-1
  Constant_-1_b02aa : Constant  Value=-1
  Constant_2.0_441df : Constant  Value=2.0
  Constant_T_dd_962be : Constant  Value=T_dd
  Constant_x_d_4e0c8 : Constant  Value=x_d
  Constant_x_dd_1c1bc : Constant  Value=x_dd
  Constant_x_dd_4ac5f : Constant  Value=x_dd
  Constant_x_dd_4b1ce : Constant  Value=x_dd
  Constant_x_dd_55ec8 : Constant  Value=x_dd
  Constant_x_dd_6580e : Constant  Value=x_dd
  Constant_x_dd_6a1fb : Constant  Value=x_dd
  Constant_x_dd_7046e : Constant  Value=x_dd
  Constant_x_dd_80348 : Constant  Value=x_dd
  Constant_x_dd_a8122 : Constant  Value=x_dd
  Constant_x_dd_f518c : Constant  Value=x_dd
  Constant_x_ddd_0bfb5 : Constant  Value=x_ddd
  Constant_x_ddd_12a34 : Constant  Value=x_ddd
  Constant_x_ddd_25d60 : Constant  Value=x_ddd
  Constant_x_ddd_3cce7 : Constant  Value=x_ddd
  Constant_x_ddd_416b4 : Constant  Value=x_ddd
  Constant_x_ddd_59f35 : Constant  Value=x_ddd
  Constant_x_ddd_73ad3 : Constant  Value=x_ddd
  Constant_x_l_08e41 : Constant  Value=x_l
  Constant_x_l_2484c : Constant  Value=x_l
  Constant_x_l_35e6c : Constant  Value=x_l
  Constant_x_l_6e949 : Constant  Value=x_l
  Constant_x_l_72ba2 : Constant  Value=x_l
  Constant_x_l_7ef37 : Constant  Value=x_l
  Constant_x_l_af262 : Constant  Value=x_l
  Constant_x_l_e1462 : Constant  Value=x_l
  Divide_0a803 : Product  Inputs=*/
  Divide_257cf : Product  Inputs=*/
  Divide_4016c : Product  Inputs=*/
  Divide_61922 : Product  Inputs=*/
  Divide_69e9a : Product  Inputs=*/
  Divide_91817 : Product  Inputs=*/
  Divide_9b901 : Product  Inputs=*/
  Divide_f1428 : Product  Inputs=*/
  Power_e79a5 : Math  Operator=pow
  Product_12174 : Product
  Product_138d6 : Product
  Product_14f80 : Product
  Product_46a0b : Product
  Product_607ed : Product
  Product_740ad : Product
  Product_82fe9 : Product
  Product_bc6ec : Product
  Product_cdf4b : Product
  Product_d8dba : Product
  Subtract_12730 : Sum  Inputs=+-
  Subtract_27243 : Sum  Inputs=+-
  Subtract_39184 : Sum  Inputs=+-
  Subtract_3c7ef : Sum  Inputs=+-
  Subtract_4a305 : Sum  Inputs=+-
  Subtract_6395f : Sum  Inputs=+-
  Subtract_7717c : Sum  Inputs=+-
  Subtract_87c82 : Sum  Inputs=+-
  Subtract_8ff4f : Sum  Inputs=+-
  Subtract_91c12 : Sum  Inputs=+-
  Subtract_c48ed : Sum  Inputs=+-
  Subtract_cf202 : Sum  Inputs=+-
  Subtract_d4767 : Sum  Inputs=+-
  Subtract_d48fc : Sum  Inputs=+-
  Subtract_dde82 : Sum  Inputs=+-
  Subtract_eae22 : Sum  Inputs=+-
  Subtract_f652f : Sum  Inputs=+-
  Subtract_f6b75 : Sum  Inputs=+-
  Subtract_fe307 : Sum  Inputs=+-
  Blockout_d_psi_fd_SG_D_1_0294b : Outport
  wires:
  State_psi_d_SG_D_1_cb963/1 -> Add_54c53/2
  Constant_x_dd_7046e/1 -> Subtract_f652f/1
  Product_14f80/1 -> Divide_4016c/1
  Subtract_4a305/1 -> Product_14f80/2
  Subtract_fe307/1 -> Product_138d6/2
  Product_12174/1 -> Product_14f80/1
  Constant_x_dd_6580e/1 -> Subtract_4a305/1
  Constant_x_l_7ef37/1 -> Subtract_cf202/2
  Constant_-1_08871/1 -> Product_12174/1
  Subtract_cf202/1 -> Product_138d6/1
  Constant_x_l_08e41/1 -> Subtract_f652f/2
  Constant_x_ddd_3cce7/1 -> Subtract_4a305/2
  State_psi_1d_SG_D_1_4f731/1 -> Product_12174/2
  Constant_x_ddd_25d60/1 -> Subtract_d48fc/1
  Constant_x_l_72ba2/1 -> Subtract_d48fc/2
  State_E_fd_SG_D_1_29de2/1 -> Subtract_87c82/1
  Divide_4016c/1 -> Add_54c53/1
  Subtract_f652f/1 -> Divide_4016c/2
  State_psi_fd_SG_D_1_e1815/1 -> Product_740ad/1
  Constant_x_ddd_416b4/1 -> Divide_69e9a/2
  Subtract_d48fc/1 -> Product_740ad/2
  Constant_x_dd_80348/1 -> Subtract_eae22/1
  Constant_x_dd_4ac5f/1 -> Subtract_f6b75/1
  State_psi_fd_SG_D_1_0848f/1 -> Subtract_87c82/2
  Constant_x_l_2484c/1 -> Subtract_eae22/2
  Product_740ad/1 -> Divide_257cf/1
  Constant_-1_b02aa/1 -> Product_82fe9/1
  Subtract_eae22/1 -> Divide_257cf/2
  Constant_x_dd_55ec8/1 -> Subtract_cf202/1
  Add_54c53/1 -> Subtract_fe307/1
  Constant_x_l_e1462/1 -> Subtract_f6b75/2
  Divide_257cf/1 -> Subtract_fe307/2
  Divide_9b901/1 -> Subtract_7717c/1
  Constant_-1_643bb/1 -> Product_d8dba/1
  State_psi_1d_SG_D_1_7ebda/1 -> Product_d8dba/2
  Constant_x_dd_f518c/1 -> Subtract_c48ed/1
  Subtract_27243/1 -> Product_82fe9/2
  Constant_x_ddd_12a34/1 -> Subtract_c48ed/2
  Product_d8dba/1 -> Product_cdf4b/1
  Constant_2.0_441df/1 -> Power_e79a5/2
  Product_cdf4b/1 -> Divide_61922/1
  Subtract_7717c/1 -> Product_46a0b/2
  Subtract_c48ed/1 -> Product_cdf4b/2
  State_psi_d_SG_D_1_ec3d5/1 -> Add_cb5e7/2
  Constant_x_dd_1c1bc/1 -> Subtract_dde82/1
  Constant_x_l_35e6c/1 -> Subtract_dde82/2
  Constant_x_dd_6a1fb/1 -> Subtract_27243/1
  Divide_69e9a/1 -> Subtract_91c12/2
  Constant_x_ddd_0bfb5/1 -> Subtract_39184/1
  Constant_x_ddd_73ad3/1 -> Subtract_27243/2
  Constant_x_l_af262/1 -> Subtract_39184/2
  Subtract_39184/1 -> Product_607ed/2
  State_psi_1d_SG_D_1_08c92/1 -> Subtract_12730/1
  Product_607ed/1 -> Divide_91817/1
  State_psi_fd_SG_D_1_d8d8e/1 -> Subtract_12730/2
  State_psi_fd_SG_D_1_d3425/1 -> Product_607ed/1
  Product_138d6/1 -> Divide_69e9a/1
  Divide_61922/1 -> Add_cb5e7/1
  Subtract_dde82/1 -> Divide_61922/2
  Constant_x_dd_4b1ce/1 -> Subtract_6395f/1
  Constant_x_l_6e949/1 -> Subtract_6395f/2
  Divide_91817/1 -> Subtract_d4767/2
  Subtract_12730/1 -> Subtract_91c12/1
  Subtract_6395f/1 -> Divide_91817/2
  Subtract_91c12/1 -> Product_bc6ec/2
  Product_82fe9/1 -> Product_bc6ec/1
  Subtract_f6b75/1 -> Power_e79a5/1
  Add_cb5e7/1 -> Subtract_d4767/1
  Product_bc6ec/1 -> Divide_9b901/1
  Power_e79a5/1 -> Divide_9b901/2
  Subtract_d4767/1 -> Divide_0a803/1
  Constant_x_ddd_59f35/1 -> Divide_0a803/2
  Constant_x_d_4e0c8/1 -> Subtract_3c7ef/1
  Constant_x_dd_a8122/1 -> Subtract_3c7ef/2
  Divide_0a803/1 -> Subtract_7717c/2
  Subtract_3c7ef/1 -> Product_46a0b/1
  Subtract_87c82/1 -> Subtract_8ff4f/1
  Product_46a0b/1 -> Subtract_8ff4f/2
  Subtract_8ff4f/1 -> Divide_f1428/1
  Constant_T_dd_962be/1 -> Divide_f1428/2
  Divide_f1428/1 -> Blockout_d_psi_fd_SG_D_1_0294b/1

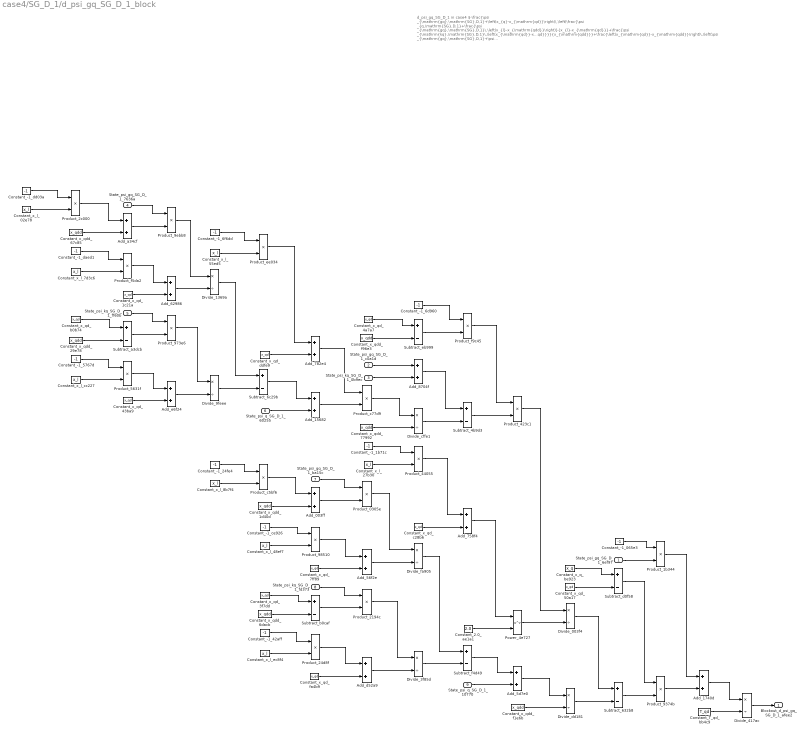
== system case4/SG_D_1/d_psi_gq_SG_D_1_block ==
  note: d_psi_gq_SG_D_1 in case4
      | $-\frac{\psi _{\mathrm{gq},\mathrm{SG},D,1}+\left(x_{q}-x_{\mathrm{qd}}\right)\,\left(\frac{\psi _{q,\mathrm{SG},D,1}+\frac{\psi _{\mathrm{gq},\mathrm{SG},D,1}\,\left(x_{l}-x_{\mathrm{qdd}}\right)}{x_{l}-x_{\mathrm{qd}}}+\frac{\psi _{\mathrm{kq},\mathrm{SG},D,1}\,\left(x_{\mathrm{qd}}-x_{\mathrm{qdd}}\right)}{x_{l}-x_{\mathrm{qd}}}}{x_{\mathrm{qdd}}}+\frac{\left(x_{\mathrm{qd}}-x_{\mathrm{qdd}}\right)\,\left(\psi _{\mathrm{gq},\mathrm{SG},D,1}+\psi _{\mathrm{kq},\mathrm{SG},D,1}+\frac{\left(x_{l}-x_{\mathrm{qd}}\right)\,\left(\psi _{q,\mathrm{SG},D,1}+\frac{\psi _{\mathrm{gq},\mathrm{SG},D,1}\,\left(x_{l}-x_{\mathrm{qdd}}\right)}{x_{l}-x_{\mathrm{qd}}}+\frac{\psi _{\mathrm{kq},\mathrm{SG},D,1}\,\left(x_{\mathrm{qd}}-x_{\mathrm{qdd}}\right)}{x_{l}-x_{\mathrm{qd}}}\right)}{x_{\mathrm{qdd}}}\right)}{{\left(x_{l}-x_{\mathrm{qd}}\right)}^2}\right)}{T_{\mathrm{qd}}}$
      | Automatically generated on 2025-10-31 19:04:24 .
  State_psi_gq_SG_D_1_6ef97 : Inport
  State_psi_gq_SG_D_1_c0a1d : Inport  Port=2
  State_psi_kq_SG_D_1_0b9ec : Inport  Port=3
  State_psi_gq_SG_D_1_7636a : Inport  Port=4
  State_psi_kq_SG_D_1_ff60b : Inport  Port=5
  State_psi_q_SG_D_1_60255 : Inport  Port=6
  State_psi_gq_SG_D_1_ba15c : Inport  Port=7
  State_psi_kq_SG_D_1_fd373 : Inport  Port=8
  State_psi_q_SG_D_1_10770 : Inport  Port=9
  Add_003ff : Sum
  Add_15682 : Sum
  Add_1740d : Sum
  Add_56f2e : Sum
  Add_5d7e0 : Sum
  Add_62986 : Sum
  Add_758f4 : Sum
  Add_782e4 : Sum
  Add_8704f : Sum
  Add_a34cf : Sum
  Add_d52a9 : Sum
  Add_e6f24 : Sum
  Constant_-1_065e3 : Constant  Value=-1
  Constant_-1_1b71c : Constant  Value=-1
  Constant_-1_24fe4 : Constant  Value=-1
  Constant_-1_42aff : Constant  Value=-1
  Constant_-1_5767d : Constant  Value=-1
  Constant_-1_6d960 : Constant  Value=-1
  Constant_-1_6f6dd : Constant  Value=-1
  Constant_-1_ce926 : Constant  Value=-1
  Constant_-1_daed1 : Constant  Value=-1
  Constant_-1_dd03a : Constant  Value=-1
  Constant_2.0_ae1a1 : Constant  Value=2.0
  Constant_T_qd_bb4c9 : Constant  Value=T_qd
  Constant_x_l_02e78 : Constant  Value=x_l
  Constant_x_l_27b30 : Constant  Value=x_l
  Constant_x_l_48ef7 : Constant  Value=x_l
  Constant_x_l_55ed5 : Constant  Value=x_l
  Constant_x_l_7d3c6 : Constant  Value=x_l
  Constant_x_l_8b7f4 : Constant  Value=x_l
  Constant_x_l_cc227 : Constant  Value=x_l
  Constant_x_l_ec8f4 : Constant  Value=x_l
  Constant_x_q_be923 : Constant  Value=x_q
  Constant_x_qd_1c21a : Constant  Value=x_qd
  Constant_x_qd_3f7dd : Constant  Value=x_qd
  Constant_x_qd_43ba9 : Constant  Value=x_qd
  Constant_x_qd_4a7a7 : Constant  Value=x_qd
  Constant_x_qd_50a17 : Constant  Value=x_qd
  Constant_x_qd_7ff89 : Constant  Value=x_qd
  Constant_x_qd_b0b74 : Constant  Value=x_qd
  Constant_x_qd_c28b6 : Constant  Value=x_qd
  Constant_x_qd_ddfe9 : Constant  Value=x_qd
  Constant_x_qd_fa4b9 : Constant  Value=x_qd
  Constant_x_qdd_1d40d : Constant  Value=x_qdd
  Constant_x_qdd_29e78 : Constant  Value=x_qdd
  Constant_x_qdd_67c85 : Constant  Value=x_qdd
  Constant_x_qdd_6dacb : Constant  Value=x_qdd
  Constant_x_qdd_77992 : Constant  Value=x_qdd
  Constant_x_qdd_f1e6b : Constant  Value=x_qdd
  Constant_x_qdd_f96e3 : Constant  Value=x_qdd
  Divide_003f4 : Product  Inputs=*/
  Divide_1369a : Product  Inputs=*/
  Divide_3f85d : Product  Inputs=*/
  Divide_417ac : Product  Inputs=*/
  Divide_9feee : Product  Inputs=*/
  Divide_cffe1 : Product  Inputs=*/
  Divide_dd181 : Product  Inputs=*/
  Divide_fa905 : Product  Inputs=*/
  Power_4e727 : Math  Operator=pow
  Product_0305e : Product
  Product_1b344 : Product
  Product_2194c : Product
  Product_24d8f : Product
  Product_2c000 : Product
  Product_423c1 : Product
  Product_44055 : Product
  Product_5631f : Product
  Product_9374b : Product
  Product_973e6 : Product
  Product_98510 : Product
  Product_9ebb8 : Product
  Product_c5bf6 : Product
  Product_c77d9 : Product
  Product_ee034 : Product
  Product_f5da2 : Product
  Product_f9c45 : Product
  Subtract_4b9d3 : Sum  Inputs=+-
  Subtract_632b8 : Sum  Inputs=+-
  Subtract_6c29b : Sum  Inputs=+-
  Subtract_a3dcb : Sum  Inputs=+-
  Subtract_b0caf : Sum  Inputs=+-
  Subtract_d0f58 : Sum  Inputs=+-
  Subtract_eb999 : Sum  Inputs=+-
  Subtract_f4d49 : Sum  Inputs=+-
  Blockout_d_psi_gq_SG_D_1_afee2 : Outport
  wires:
  State_psi_gq_SG_D_1_7636a/1 -> Product_9ebb8/1
  Constant_-1_daed1/1 -> Product_f5da2/1
  Divide_1369a/1 -> Subtract_6c29b/1
  Add_62986/1 -> Divide_1369a/2
  Product_2c000/1 -> Add_a34cf/1
  Constant_x_qd_ddfe9/1 -> Add_782e4/2
  Constant_-1_dd03a/1 -> Product_2c000/1
  Constant_x_qdd_67c85/1 -> Add_a34cf/2
  Constant_x_l_7d3c6/1 -> Product_f5da2/2
  Constant_x_l_02e78/1 -> Product_2c000/2
  Constant_-1_5767d/1 -> Product_5631f/1
  Constant_x_qd_b0b74/1 -> Subtract_a3dcb/1
  Constant_x_qdd_77992/1 -> Divide_cffe1/2
  Constant_x_l_cc227/1 -> Product_5631f/2
  Constant_x_qdd_29e78/1 -> Subtract_a3dcb/2
  Subtract_6c29b/1 -> Add_15682/1
  Add_a34cf/1 -> Product_9ebb8/2
  Product_9ebb8/1 -> Divide_1369a/1
  Product_f5da2/1 -> Add_62986/1
  Constant_x_qd_1c21a/1 -> Add_62986/2
  State_psi_kq_SG_D_1_ff60b/1 -> Product_973e6/1
  Product_5631f/1 -> Add_e6f24/1
  Subtract_a3dcb/1 -> Product_973e6/2
  Constant_x_qd_43ba9/1 -> Add_e6f24/2
  Product_973e6/1 -> Divide_9feee/1
  Add_e6f24/1 -> Divide_9feee/2
  Constant_-1_6d960/1 -> Product_f9c45/1
  Constant_-1_6f6dd/1 -> Product_ee034/1
  Add_56f2e/1 -> Divide_fa905/2
  Product_24d8f/1 -> Add_d52a9/1
  Subtract_b0caf/1 -> Product_2194c/2
  Constant_x_l_55ed5/1 -> Product_ee034/2
  Divide_9feee/1 -> Subtract_6c29b/2
  Subtract_d0f58/1 -> Product_9374b/1
  Constant_-1_1b71c/1 -> Product_44055/1
  Constant_-1_24fe4/1 -> Product_c5bf6/1
  Constant_x_l_27b30/1 -> Product_44055/2
  Constant_x_l_8b7f4/1 -> Product_c5bf6/2
  Constant_x_qd_7ff89/1 -> Add_56f2e/2
  Product_ee034/1 -> Add_782e4/1
  State_psi_q_SG_D_1_60255/1 -> Add_15682/2
  Product_c5bf6/1 -> Add_003ff/1
  Constant_x_qdd_1d40d/1 -> Add_003ff/2
  Constant_-1_ce926/1 -> Product_98510/1
  Constant_x_qd_fa4b9/1 -> Add_d52a9/2
  Add_782e4/1 -> Product_c77d9/1
  Constant_x_l_48ef7/1 -> Product_98510/2
  Constant_-1_42aff/1 -> Product_24d8f/1
  Constant_x_qd_3f7dd/1 -> Subtract_b0caf/1
  Product_c77d9/1 -> Divide_cffe1/1
  Constant_x_l_ec8f4/1 -> Product_24d8f/2
  Divide_003f4/1 -> Subtract_632b8/1
  Constant_x_qdd_6dacb/1 -> Subtract_b0caf/2
  Add_15682/1 -> Product_c77d9/2
  State_psi_gq_SG_D_1_ba15c/1 -> Product_0305e/1
  Add_003ff/1 -> Product_0305e/2
  Product_98510/1 -> Add_56f2e/1
  State_psi_kq_SG_D_1_fd373/1 -> Product_2194c/1
  Add_d52a9/1 -> Divide_3f85d/2
  State_psi_gq_SG_D_1_c0a1d/1 -> Add_8704f/1
  Constant_x_qd_4a7a7/1 -> Subtract_eb999/1
  Constant_x_qdd_f96e3/1 -> Subtract_eb999/2
  Product_2194c/1 -> Divide_3f85d/1
  State_psi_kq_SG_D_1_0b9ec/1 -> Add_8704f/2
  Product_0305e/1 -> Divide_fa905/1
  Subtract_eb999/1 -> Product_f9c45/2
  Add_8704f/1 -> Subtract_4b9d3/1
  Divide_cffe1/1 -> Subtract_4b9d3/2
  Product_44055/1 -> Add_758f4/1
  Constant_x_qd_c28b6/1 -> Add_758f4/2
  Divide_fa905/1 -> Subtract_f4d49/1
  Divide_3f85d/1 -> Subtract_f4d49/2
  Product_f9c45/1 -> Product_423c1/1
  Subtract_4b9d3/1 -> Product_423c1/2
  Add_758f4/1 -> Power_4e727/1
  Constant_2.0_ae1a1/1 -> Power_4e727/2
  Subtract_f4d49/1 -> Add_5d7e0/1
  State_psi_q_SG_D_1_10770/1 -> Add_5d7e0/2
  Product_423c1/1 -> Divide_003f4/1
  Power_4e727/1 -> Divide_003f4/2
  Add_5d7e0/1 -> Divide_dd181/1
  Constant_x_qdd_f1e6b/1 -> Divide_dd181/2
  Constant_x_q_be923/1 -> Subtract_d0f58/1
  Constant_x_qd_50a17/1 -> Subtract_d0f58/2
  Divide_dd181/1 -> Subtract_632b8/2
  Constant_-1_065e3/1 -> Product_1b344/1
  State_psi_gq_SG_D_1_6ef97/1 -> Product_1b344/2
  Subtract_632b8/1 -> Product_9374b/2
  Product_1b344/1 -> Add_1740d/1
  Product_9374b/1 -> Add_1740d/2
  Add_1740d/1 -> Divide_417ac/1
  Constant_T_qd_bb4c9/1 -> Divide_417ac/2
  Divide_417ac/1 -> Blockout_d_psi_gq_SG_D_1_afee2/1
